simulink model "Disparity_CT"  (R2021a)
settings: Solver=VariableStepAuto  StartTime=0.0  StopTime=Ts_480p*2  RelTol=1e-3
InitFcn:
  | Ts = 1e-3;
  | Ts_240p = 402*324*Ts;
  | Ts_480p = 525*800*Ts;
undefined symbols (not defined in the file or in its folder): gray
libraries: hdlsllib x7, simulink x7, visionhdlio x2, dspvision x1
settings Model: Creator=user  LastModifiedBy=user
settings OptimizationCC: BlockReduction=off  ConditionallyExecuteInputs=off  DefaultParameterBehavior=Inlined
settings DebuggingCC: AlgebraicLoopMsg=error
settings HardwareCC: ProdBitPerPointer=32  ProdBitPerSizeT=32  ProdBitPerPtrDiffT=32  ProdLargestAtomicFloat=None  ProdIntDivRoundTo=Undefined  ProdEndianess=Unspecified  ProdWordSize=32  ProdHWDeviceType=ASIC/FPGA->ASIC/FPGA  TargetBitPerPointer=64  TargetBitPerSizeT=64  TargetBitPerPtrDiffT=64  TargetLongLongMode=on  TargetIntDivRoundTo=Zero  TargetEndianess=LittleEndian  TargetWordSize=64  TargetHWDeviceType=Custom Processor->MATLAB Host Computer  ProdEqTarget=off

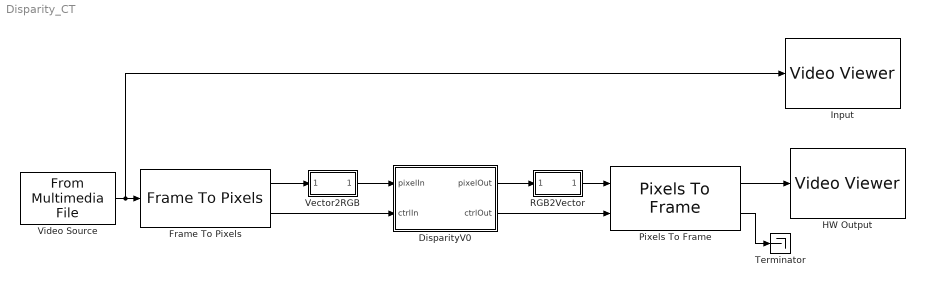
== system Disparity_CT ==
  DisparityV0 : Subsystem  TreatAsAtomicUnit=on
  Frame To Pixels : visionhdlio/Frame To Pixels  NumComponents=3  NumPixels=1  VideoFormat=480p  ActivePixelsPerLine=32  ActiveVideoLines=18  TotalPixelsPerLine=42  TotalVideoLines=28  StartingActiveLine=6  FrontPorch=5  SampleTime=0
      settings: SourceProductBaseCode=VT
  HW Output : VideoViewer  colormapValue=gray(256)  FigPos=[146 735 588 436]
  Input : VideoViewer  colormapValue=gray(256)  FigPos=[86 739 588 436]
  Pixels To Frame : visionhdlio/Pixels To Frame  NumComponents=3  NumPixels=1  VideoFormat=480p  ActivePixelsPerLine=32  ActiveVideoLines=18  TotalPixelsPerLine=42  TotalVideoLines=28
      settings: SourceProductBaseCode=VT
  RGB2Vector : Subsystem
  Terminator : Terminator
  Vector2RGB : Subsystem
  Video Source : dspvision/From Multimedia File  inputFilename=D:\Work\XilFPGAdev\Custom_IP_Cores\MathworksHDLCoder\Disparity\stereoTestimg_01_480p.bmp  readRange=[1 Inf]  loop=on  numPlays=inf  outputStreams=Video only  videoDataType=uint8  audioDataType=int16  inheritSampleTime=off  userDefinedSampleTime=Ts_480p  noAudioOutput=off  isIntensityVideo=off  fourcc=RGB  colorVideoFormat=One multidimensional signal  outputEOF=off  dataOrg=Column-major  audioFrameSize=1024  computeAudioFrameSize=off  outSamplingMode=Sample based
  wires:
  Vector2RGB/1(RGB) -> DisparityV0/1(pixelIn)
  RGB2Vector/1(RGBVector) -> Pixels To Frame/1
  Frame To Pixels/1 -> Vector2RGB/1(RGBVector)
  Frame To Pixels/2 -> DisparityV0/2(ctrlIn)
  Pixels To Frame/1 -> HW Output/1
  Pixels To Frame/2 -> Terminator/1
  Video Source/1 -> Input/1, Frame To Pixels/1
  DisparityV0/1(pixelOut) -> RGB2Vector/1(RGB)
  DisparityV0/2(ctrlOut) -> Pixels To Frame/2

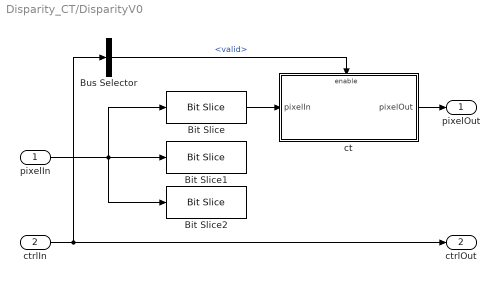
== system Disparity_CT/DisparityV0 ==
  pixelIn : Inport
  ctrlIn : Inport  Port=2
  Bit Slice : hdlsllib/Logic and Bit Operations/Bit Slice  lidx=23  ridx=16
      settings: SourceProductBaseCode=SL
  Bit Slice1 : hdlsllib/Logic and Bit Operations/Bit Slice  lidx=15  ridx=8
      settings: SourceProductBaseCode=SL
  Bit Slice2 : hdlsllib/Logic and Bit Operations/Bit Slice  lidx=7  ridx=0
      settings: SourceProductBaseCode=SL
  Bus Selector : BusSelector  OutputSignals=valid
  ct : Subsystem
  pixelOut : Outport
  ctrlOut : Outport  Port=2  VectorParamsAs1DForOutWhenUnconnected=off
  wires:
  ctrlIn/1 -> ctrlOut/1, Bus Selector/1
  Bit Slice/1 -> ct/1(pixelIn)
  Bus Selector/1 -> ct/Enable  "<valid>"
  pixelIn/1 -> Bit Slice2/1, Bit Slice1/1, Bit Slice/1
  ct/1(pixelOut) -> pixelOut/1

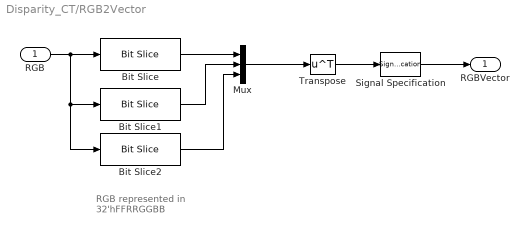
== system Disparity_CT/RGB2Vector ==
  note: RGB represented in
      | 32'hFFRRGGBB
  RGB : Inport
  Bit Slice : hdlsllib/Logic and Bit Operations/Bit Slice  lidx=23  ridx=16
      settings: SourceProductBaseCode=SL
  Bit Slice1 : hdlsllib/Logic and Bit Operations/Bit Slice  lidx=15  ridx=8
      settings: SourceProductBaseCode=SL
  Bit Slice2 : hdlsllib/Logic and Bit Operations/Bit Slice  lidx=7  ridx=0
      settings: SourceProductBaseCode=SL
  Mux : Mux  Inputs=3
  Signal Specification : SignalSpecification
  Transpose : Math  Operator=transpose  SignedPower=on  SaturateOnIntegerOverflow=on
  RGBVector : Outport  VectorParamsAs1DForOutWhenUnconnected=off
  wires:
  Mux/1 -> Transpose/1
  Bit Slice/1 -> Mux/1
  Bit Slice2/1 -> Mux/3
  Bit Slice1/1 -> Mux/2
  RGB/1 -> Bit Slice2/1, Bit Slice1/1, Bit Slice/1
  Transpose/1 -> Signal Specification/1
  Signal Specification/1 -> RGBVector/1

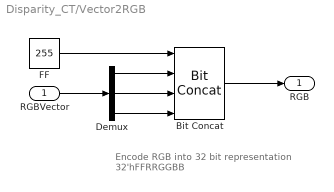
== system Disparity_CT/Vector2RGB ==
  note: Encode RGB into 32 bit representation
      | 32'hFFRRGGBB
  RGBVector : Inport
  Bit Concat : hdlsllib/Logic and Bit Operations/Bit Concat  numInputs=4
  Demux : Demux  Outputs=3
  FF : Constant  Value=255  OutDataTypeStr=uint8  SampleTime=Ts
  RGB : Outport  VectorParamsAs1DForOutWhenUnconnected=off
  wires:
  Bit Concat/1 -> RGB/1
  RGBVector/1 -> Demux/1
  FF/1 -> Bit Concat/1
  Demux/1 -> Bit Concat/2
  Demux/2 -> Bit Concat/3
  Demux/3 -> Bit Concat/4

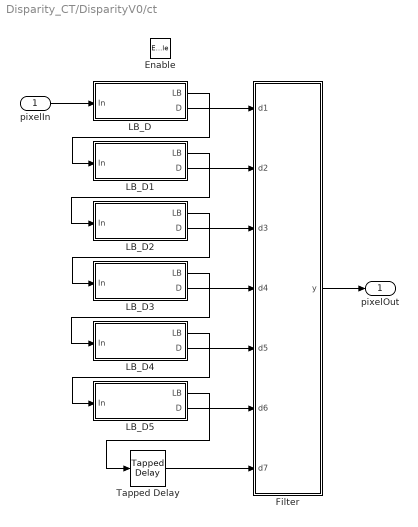
== system Disparity_CT/DisparityV0/ct ==
  pixelIn : Inport
  Enable : EnablePort
  Filter : MATLAB Function  TreatAsAtomicUnit=on
  LB_D : Subsystem
  LB_D1 : Subsystem
  LB_D2 : Subsystem
  LB_D3 : Subsystem
  LB_D4 : Subsystem
  LB_D5 : Subsystem
  Tapped Delay : simulink/Discrete/Tapped Delay  vinit=0.0  samptime=-1  NumDelays=8  DelayOrder=Oldest  includeCurrent=on
  pixelOut : Outport  InitialOutput=0
  wires:
  Filter/1(y) -> pixelOut/1
  pixelIn/1 -> LB_D/1(In)
  LB_D/1(LB) -> LB_D1/1(In)
  LB_D2/1(LB) -> LB_D3/1(In)
  LB_D1/1(LB) -> LB_D2/1(In)
  LB_D5/1(LB) -> Tapped Delay/1
  LB_D4/1(LB) -> LB_D5/1(In)
  LB_D3/1(LB) -> LB_D4/1(In)
  LB_D/2(D) -> Filter/1(d1)
  LB_D1/2(D) -> Filter/2(d2)
  LB_D2/2(D) -> Filter/3(d3)
  LB_D3/2(D) -> Filter/4(d4)
  LB_D4/2(D) -> Filter/5(d5)
  LB_D5/2(D) -> Filter/6(d6)
  Tapped Delay/1 -> Filter/7(d7)

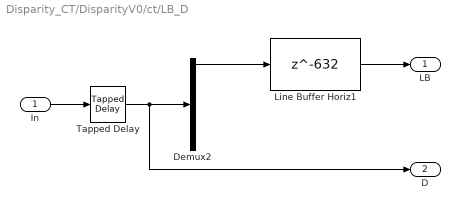
== system Disparity_CT/DisparityV0/ct/LB_D ==
  In : Inport
  Demux2 : Demux  Outputs=5
      settings: DisplayOption=none
  Line Buffer Horiz1 : Delay  DelayLength=632  InitialCondition=0
  Tapped Delay : simulink/Discrete/Tapped Delay  vinit=0.0  samptime=-1  NumDelays=8  DelayOrder=Oldest  includeCurrent=on
  LB : Outport
  D : Outport  Port=2
  wires:
  Line Buffer Horiz1/1 -> LB/1
  Tapped Delay/1 -> D/1, Demux2/1
  Demux2/1 -> Line Buffer Horiz1/1
  In/1 -> Tapped Delay/1

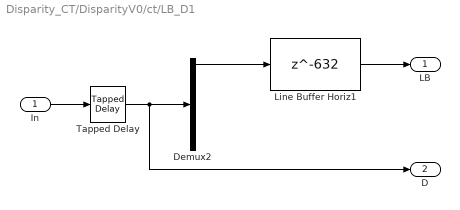
== system Disparity_CT/DisparityV0/ct/LB_D1 ==
  In : Inport
  Demux2 : Demux  Outputs=5
      settings: DisplayOption=none
  Line Buffer Horiz1 : Delay  DelayLength=632  InitialCondition=0
  Tapped Delay : simulink/Discrete/Tapped Delay  vinit=0.0  samptime=-1  NumDelays=8  DelayOrder=Oldest  includeCurrent=on
  LB : Outport
  D : Outport  Port=2
  wires:
  Line Buffer Horiz1/1 -> LB/1
  Tapped Delay/1 -> D/1, Demux2/1
  Demux2/1 -> Line Buffer Horiz1/1
  In/1 -> Tapped Delay/1

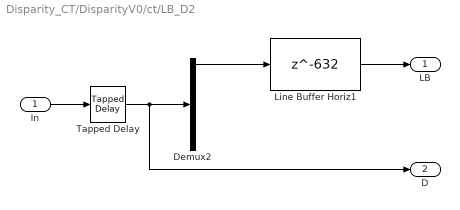
== system Disparity_CT/DisparityV0/ct/LB_D2 ==
  In : Inport
  Demux2 : Demux  Outputs=5
      settings: DisplayOption=none
  Line Buffer Horiz1 : Delay  DelayLength=632  InitialCondition=0
  Tapped Delay : simulink/Discrete/Tapped Delay  vinit=0.0  samptime=-1  NumDelays=8  DelayOrder=Oldest  includeCurrent=on
  LB : Outport
  D : Outport  Port=2
  wires:
  Line Buffer Horiz1/1 -> LB/1
  Tapped Delay/1 -> D/1, Demux2/1
  Demux2/1 -> Line Buffer Horiz1/1
  In/1 -> Tapped Delay/1

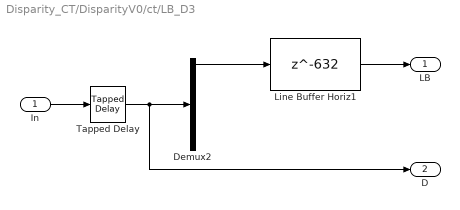
== system Disparity_CT/DisparityV0/ct/LB_D3 ==
  In : Inport
  Demux2 : Demux  Outputs=5
      settings: DisplayOption=none
  Line Buffer Horiz1 : Delay  DelayLength=632  InitialCondition=0
  Tapped Delay : simulink/Discrete/Tapped Delay  vinit=0.0  samptime=-1  NumDelays=8  DelayOrder=Oldest  includeCurrent=on
  LB : Outport
  D : Outport  Port=2
  wires:
  Line Buffer Horiz1/1 -> LB/1
  Tapped Delay/1 -> D/1, Demux2/1
  Demux2/1 -> Line Buffer Horiz1/1
  In/1 -> Tapped Delay/1

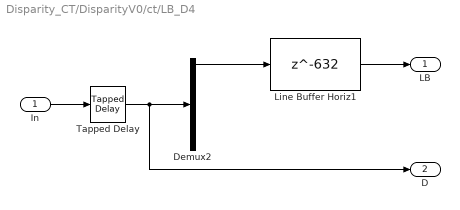
== system Disparity_CT/DisparityV0/ct/LB_D4 ==
  In : Inport
  Demux2 : Demux  Outputs=5
      settings: DisplayOption=none
  Line Buffer Horiz1 : Delay  DelayLength=632  InitialCondition=0
  Tapped Delay : simulink/Discrete/Tapped Delay  vinit=0.0  samptime=-1  NumDelays=8  DelayOrder=Oldest  includeCurrent=on
  LB : Outport
  D : Outport  Port=2
  wires:
  Line Buffer Horiz1/1 -> LB/1
  Tapped Delay/1 -> D/1, Demux2/1
  Demux2/1 -> Line Buffer Horiz1/1
  In/1 -> Tapped Delay/1

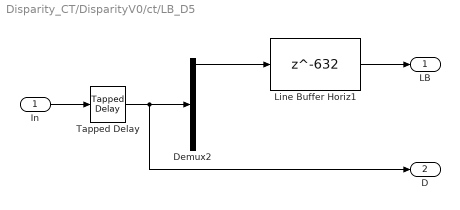
== system Disparity_CT/DisparityV0/ct/LB_D5 ==
  In : Inport
  Demux2 : Demux  Outputs=5
      settings: DisplayOption=none
  Line Buffer Horiz1 : Delay  DelayLength=632  InitialCondition=0
  Tapped Delay : simulink/Discrete/Tapped Delay  vinit=0.0  samptime=-1  NumDelays=8  DelayOrder=Oldest  includeCurrent=on
  LB : Outport
  D : Outport  Port=2
  wires:
  Line Buffer Horiz1/1 -> LB/1
  Tapped Delay/1 -> D/1, Demux2/1
  Demux2/1 -> Line Buffer Horiz1/1
  In/1 -> Tapped Delay/1

== matlab function Disparity_CT/DisparityV0/ct/Filter ==
  data: d1 input; y output; d2 input; d3 input; d4 input; d5 input; d6 input; d7 input
function y = fcn(d1,d2,d3,d4,d5,d6,d7)
d = [d1,d2,d3,d4,d5,d6,d7]'; %7x9 matrix
d = fliplr(d);
% d = fi(d,0,8,0);

c1 = d(7,9)>d(1,1);
c2 = d(7,8)>d(1,2);
c3 = d(7,7)>d(1,3);
c4 = d(7,6)>d(1,4);
c5 = d(7,5)>d(1,5);
c6 = d(7,4)>d(1,6);
c7 = d(7,3)>d(1,7);
c8 = d(7,2)>d(1,8);
c9 = d(7,1)>d(1,9);
c10 = d(6,9)>d(2,1);
c11 = d(6,8)>d(2,2);
c12 = d(6,7)>d(2,3);
c13 = d(6,6)>d(2,4);
c14 = d(6,5)>d(2,5);
c15 = d(6,4)>d(2,6);
c16 = d(6,3)>d(2,7);
c17 = d(6,2)>d(2,8);
c18 = d(6,1)>d(2,9);
c19 = d(5,9)>d(3,1);
c20 = d(5,8)>d(3,2);
c21 = d(5,7)>d(3,3);
c22 = d(5,6)>d(3,4);
c23 = d(5,5)>d(3,5);
c24 = d(5,4)>d(3,6);
c25 = d(5,3)>d(3,7);
c26 = d(5,2)>d(3,8);
c27 = d(5,1)>d(3,9);
c28 = d(4,9)>d(4,1);
c29 = d(4,8)>d(4,2);
c30 = d(4,7)>d(4,3);
c31 = d(4,6)>d(4,4);

c1 = fi(c1,0,1,0);
c2 = fi(c2,0,1,0);
c3 = fi(c3,0,1,0);
c4 = fi(c4,0,1,0);
c5 = fi(c5,0,1,0);
c6 = fi(c6,0,1,0);
c7 = fi(c7,0,1,0);
c8 = fi(c8,0,1,0);
c9 = fi(c9,0,1,0);
c10 = fi(c10,0,1,0);
c11 = fi(c11,0,1,0);
c12 = fi(c12,0,1,0);
c13 = fi(c13,0,1,0);
c14 = fi(c14,0,1,0);
c15 = fi(c15,0,1,0);
c16 = fi(c16,0,1,0);
c17 = fi(c17,0,1,0);
c18 = fi(c18,0,1,0);
c19 = fi(c19,0,1,0);
c20 = fi(c20,0,1,0);
c21 = fi(c21,0,1,0);
c22 = fi(c22,0,1,0);
c23 = fi(c23,0,1,0);
c24 = fi(c24,0,1,0);
c25 = fi(c25,0,1,0);
c26 = fi(c26,0,1,0);
c27 = fi(c27,0,1,0);
c28 = fi(c28,0,1,0);
c29 = fi(c29,0,1,0);
c30 = fi(c30,0,1,0);
c31 = fi(c31,0,1,0);

y = bitconcat(c1,c2,c3,c4,c5,c6,c7,c8,c9,c10,c11,c12,c13,c14,c15,c16,c17,c18,c19,c20,c21,c22,c23,c24,c25,c26,c27,c28,c29,c30,c31,fi(0,0,1,0));
